simulink model "network_2"  (R2018a)
settings: Solver=VariableStepAuto  StartTime=0.0  StopTime=10.0  RelTol=1e-3
libraries: powerlib x43, fl_lib x2, elec_lib x1
settings Model: Creator=Sadat Zubin Shah  LastModifiedBy=Sadat Zubin Shah

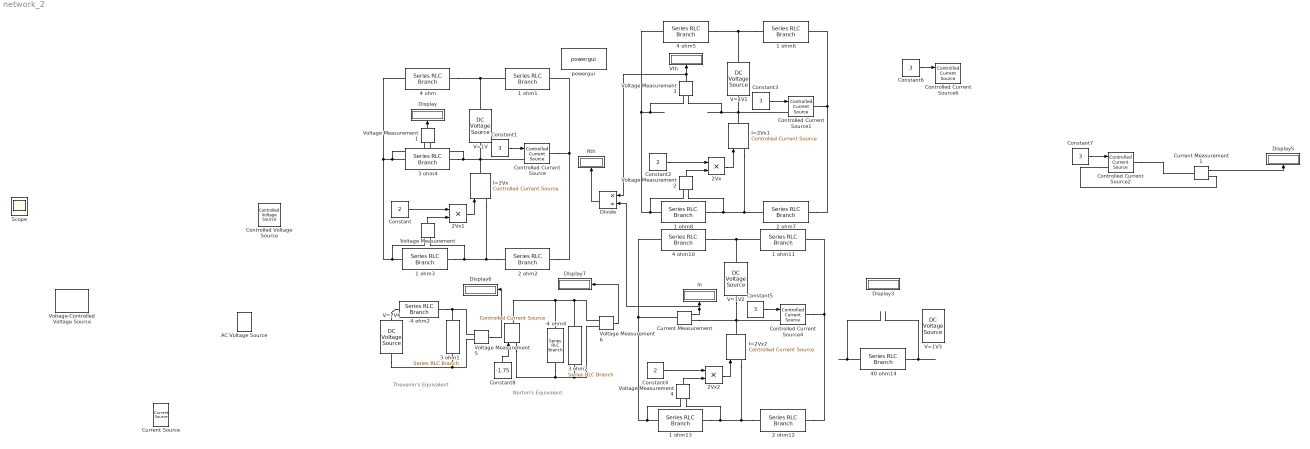
== system network_2 ==
  note: Norton's Equivalent
  note: Thevenin's Equivalent
  " " : powerlib/Electrical Sources/Controlled Current Source  Initialize=off  Source_Type=AC  Amplitude=0  Phase=0  Frequency=0  Measurements=None
  -4 ohm2 : powerlib/Elements/Series RLC Branch  LConnTagsString=__new0  RConnTagsString=__new0  BranchType=R  Resistance=-4  Inductance=1e-3  SetiL0=off  InitialCurrent=0  Capacitance=1e-6  Setx0=off  InitialVoltage=0  Measurements=None
  -4 ohm4 : powerlib/Elements/Series RLC Branch  LConnTagsString=__new0  RConnTagsString=__new0  BranchType=R  Resistance=-4  Inductance=1e-3  SetiL0=off  InitialCurrent=0  Capacitance=1e-6  Setx0=off  InitialVoltage=0  Measurements=None
  1 ohm{1,3,6,8,11,13} (6 alike) : powerlib/Elements/Series RLC Branch  LConnTagsString=__new0  RConnTagsString=__new0  BranchType=R  Resistance=1  Inductance=1e-3  SetiL0=off  InitialCurrent=0  Capacitance=1e-6  Setx0=off  InitialVoltage=0  Measurements=None
  2 ohm12 : powerlib/Elements/Series RLC Branch  LConnTagsString=__new0  RConnTagsString=__new0  BranchType=R  Resistance=2  Inductance=1e-3  SetiL0=off  InitialCurrent=0  Capacitance=1e-6  Setx0=off  InitialVoltage=0  Measurements=None
  2 ohm2 : powerlib/Elements/Series RLC Branch  LConnTagsString=__new0  RConnTagsString=__new0  BranchType=R  Resistance=2  Inductance=1e-3  SetiL0=off  InitialCurrent=0  Capacitance=1e-6  Setx0=off  InitialVoltage=0  Measurements=None
  2 ohm7 : powerlib/Elements/Series RLC Branch  LConnTagsString=__new0  RConnTagsString=__new0  BranchType=R  Resistance=2  Inductance=1e-3  SetiL0=off  InitialCurrent=0  Capacitance=1e-6  Setx0=off  InitialVoltage=0  Measurements=None
  2Vx : Product
  2Vx1 : Product
  2Vx2 : Product
  3 ohm1 : powerlib/Elements/Series RLC Branch  LConnTagsString=__new0  RConnTagsString=__new0  BranchType=R  Resistance=3  Inductance=1e-3  SetiL0=off  InitialCurrent=0  Capacitance=1e-6  Setx0=off  InitialVoltage=0  Measurements=None
  3 ohm2 : powerlib/Elements/Series RLC Branch  LConnTagsString=__new0  RConnTagsString=__new0  BranchType=R  Resistance=3  Inductance=1e-3  SetiL0=off  InitialCurrent=0  Capacitance=1e-6  Setx0=off  InitialVoltage=0  Measurements=None
  3 ohm4 : powerlib/Elements/Series RLC Branch  LConnTagsString=__new0  RConnTagsString=__new0  BranchType=R  Resistance=3  Inductance=1e-3  SetiL0=off  InitialCurrent=0  Capacitance=1e-6  Setx0=off  InitialVoltage=0  Measurements=None
  4 ohm : powerlib/Elements/Series RLC Branch  LConnTagsString=__new0  RConnTagsString=__new0  BranchType=R  Resistance=4  Inductance=1e-3  SetiL0=off  InitialCurrent=0  Capacitance=1e-6  Setx0=off  InitialVoltage=0  Measurements=None
  4 ohm10 : powerlib/Elements/Series RLC Branch  LConnTagsString=__new0  RConnTagsString=__new0  BranchType=R  Resistance=4  Inductance=1e-3  SetiL0=off  InitialCurrent=0  Capacitance=1e-6  Setx0=off  InitialVoltage=0  Measurements=None
  4 ohm5 : powerlib/Elements/Series RLC Branch  LConnTagsString=__new0  RConnTagsString=__new0  BranchType=R  Resistance=4  Inductance=1e-3  SetiL0=off  InitialCurrent=0  Capacitance=1e-6  Setx0=off  InitialVoltage=0  Measurements=None
  40 ohm14 : powerlib/Elements/Series RLC Branch  LConnTagsString=__new0  RConnTagsString=__new0  BranchType=R  Resistance=3  Inductance=1e-3  SetiL0=off  InitialCurrent=0  Capacitance=1e-6  Setx0=off  InitialVoltage=0  Measurements=None
  AC Voltage Source : powerlib/Electrical Sources/AC Voltage Source  Amplitude=100  Phase=0  Frequency=60  SampleTime=0  Measurements=None  BusType=swing  Pref=10e3  Qref=0  Qmin=-inf  Qmax=+inf
  Constant : Constant  Value=2
  Constant{1,3,5..7} (5 alike) : Constant  Value=3
  Constant2 : Constant  Value=2
  Constant4 : Constant  Value=2
  Constant8 : Constant  Value=-1.75
  Controlled Current Source{,1..2,4,6} (5 alike) : powerlib/Electrical Sources/Controlled Current Source  Initialize=off  Source_Type=AC  Amplitude=0  Phase=0  Frequency=0  Measurements=None
  Controlled Voltage Source : fl_lib/Electrical/Electrical Sources/Controlled Voltage Source
  Current Measurement : powerlib/Measurements/Current Measurement  PhasorSimulation=off  OutputType=Complex  PSBequivalent=0
  Current Measurement1 : powerlib/Measurements/Current Measurement  PhasorSimulation=off  OutputType=Complex  PSBequivalent=0
  Current Source : elec_lib/Sources/Current Source  dc_current=0 A  ac_current=0 A  ac_shift=0 rad  ac_frequency=60 Hz  noise_mode=0  PSD=0 A^2/Hz  repeatability=1  auto_seed=3499211588  user_seed=0  sample_time=1e-3 s  i_specify=off  i_priority=None  i=0 A  i_nominal_specify=off  i_nominal_unit=A  i_nominal_value=1  v_specify=off  v_priority=None  v=0 V  v_nominal_specify=off  v_nominal_unit=V  v_nominal_value=1
      settings: SourceProductName=Simscape Electronics  SourceProductBaseCode=SN
  Display{,3,5..7} (5 alike) : Display
  Divide : Product  Inputs=*/
  I=2Vx : powerlib/Electrical Sources/Controlled Current Source  Initialize=off  Source_Type=AC  Amplitude=0  Phase=0  Frequency=0  Measurements=None
  I=2Vx1 : powerlib/Electrical Sources/Controlled Current Source  Initialize=off  Source_Type=AC  Amplitude=0  Phase=0  Frequency=0  Measurements=None
  I=2Vx2 : powerlib/Electrical Sources/Controlled Current Source  Initialize=off  Source_Type=AC  Amplitude=0  Phase=0  Frequency=0  Measurements=None
  In : Display
  Rth : Display
  Scope : Scope
  V=1V : powerlib/Electrical Sources/DC Voltage Source  Amplitude=1  Measurements=None
  V=1V1 : powerlib/Electrical Sources/DC Voltage Source  Amplitude=1  Measurements=None
  V=1V2 : powerlib/Electrical Sources/DC Voltage Source  Amplitude=1  Measurements=None
  V=1V3 : powerlib/Electrical Sources/DC Voltage Source  Amplitude=10  Measurements=None
  V=7V4 : powerlib/Electrical Sources/DC Voltage Source  Amplitude=7  Measurements=None
  Voltage Measurement{,1..6} (7 alike) : powerlib/Measurements/Voltage Measurement  PhasorSimulation=off  OutputType=Complex  PSBequivalent=0
  Voltage-Controlled Voltage Source : fl_lib/Electrical/Electrical Sources/Voltage-Controlled Voltage Source  K=1  v1_specify=off  v1_priority=None  v1=0 V  v1_nominal_specify=off  v1_nominal_unit=V  v1_nominal_value=1  v2_specify=off  v2_priority=None  v2=0 V  v2_nominal_specify=off  v2_nominal_unit=V  v2_nominal_value=1
      settings: SourceProductName=Simscape  SourceProductBaseCode=SS
  Vth : Display
  powergui : powerlib/powergui  Priority=1  SimulationMode=Continuous  SampleTime=50e-6  frequency=60  Iterations=50  frequencyindice=0  Pbase=100e6  ErrMax=1e-4  UnitsV=kV  UnitsW=MW  buscounter=0  FunctionMessages=off  echomessages=off  EnableUseOfTLC=off  CurrentSourceSwitches=off  DisableSnubberDevices=off  DisableRonSwitches=off  DisableVfSwitches=off  DisplayEquations=off  SolverType=Tustin/Backward Euler (TBE)  Interpol=off  ExternalGateDelay=off  methode=off  Ts=100  x0status=blocks  SPID=on  SwTol=0  HookPort=off  RestoreLinks=warning  ResistiveCurrentMeasurement=off  Frange=[0:2:500]  Ylog=off  Xlog=off  ShowGrid=on  save=off  variable=ZData  structure=0  ZoomFFT=off  StartTime=0.0  cycles=1  DisplayStyle=1  fundamental=60  FreqAxis=off  MaxFrequency=1000  frequencyindicesteady=1  RmsSteady=1  display=off
  wires:
  Voltage Measurement/1 -> 2Vx1/2
  Constant/1 -> 2Vx1/1
  2Vx1/1 -> I=2Vx/1
  Constant1/1 -> Controlled Current Source/1
  Voltage Measurement1/1 -> Display/1
  Voltage Measurement3/1 -> Vth/1, Divide/1
  2Vx/1 -> I=2Vx1/1
  Constant2/1 -> 2Vx/1
  Voltage Measurement2/1 -> 2Vx/2
  Voltage Measurement4/1 -> 2Vx2/2
  Constant4/1 -> 2Vx2/1
  2Vx2/1 -> I=2Vx2/1
  Constant5/1 -> Controlled Current Source4/1
  Constant6/1 -> Controlled Current Source6/1
  ? -> Display3/1
  Current Measurement/1 -> Divide/2, In/1
  Divide/1 -> Rth/1
  Constant3/1 -> Controlled Current Source1/1
  Constant7/1 -> Controlled Current Source2/1
  Current Measurement1/1 -> Display5/1
  Voltage Measurement5/1 -> Display6/1
  Constant8/1 -> " "/1
  Voltage Measurement6/1 -> Display7/1
  connections:
  3 ohm4/RConn1 -- Voltage Measurement1/LConn2 -- I=2Vx/RConn1 -- Controlled Current Source/LConn1 -- V=1V/LConn1
  2 ohm2/RConn1 -- Controlled Current Source/RConn1 -- 1 ohm1/RConn1
  2 ohm2/LConn1 -- Voltage Measurement/LConn2 -- 1 ohm3/RConn1 -- I=2Vx/LConn1
  1 ohm3/LConn1 -- Voltage Measurement/LConn1 -- 4 ohm/LConn1 -- Voltage Measurement1/LConn1 -- 3 ohm4/LConn1
  4 ohm/RConn1 -- 1 ohm1/LConn1 -- V=1V/RConn1
  I=2Vx1/RConn1 -- V=1V1/LConn1 -- Controlled Current Source1/LConn1 -- Voltage Measurement3/LConn2
  Voltage Measurement2/LConn2 -- 1 ohm8/RConn1 -- I=2Vx1/LConn1 -- 2 ohm7/LConn1
  Voltage Measurement2/LConn1 -- 1 ohm8/LConn1 -- Voltage Measurement3/LConn1 -- 4 ohm5/LConn1
  1 ohm6/LConn1 -- V=1V1/RConn1 -- 4 ohm5/RConn1
  1 ohm11/RConn1 -- 2 ohm12/RConn1 -- Controlled Current Source4/RConn1
  2 ohm12/LConn1 -- Voltage Measurement4/LConn2 -- 1 ohm13/RConn1 -- I=2Vx2/LConn1
  1 ohm13/LConn1 -- Current Measurement/LConn1 -- 4 ohm10/LConn1 -- Voltage Measurement4/LConn1
  Controlled Current Source4/LConn1 -- Current Measurement/RConn1 -- V=1V2/LConn1 -- I=2Vx2/RConn1
  40 ohm14/RConn1 -- ?
  40 ohm14/LConn1 -- ?
  2 ohm7/RConn1 -- Controlled Current Source1/RConn1 -- 1 ohm6/RConn1
  4 ohm10/RConn1 -- V=1V2/RConn1 -- 1 ohm11/LConn1
  Controlled Current Source2/RConn1 -- Current Measurement1/LConn1
  Current Measurement1/RConn1 -- Controlled Current Source2/LConn1
  V=7V4/RConn1 -- -4 ohm2/LConn1
  -4 ohm2/RConn1 -- Voltage Measurement5/LConn1 -- 3 ohm1/LConn1
  V=7V4/LConn1 -- Voltage Measurement5/LConn2 -- 3 ohm1/RConn1
  Voltage Measurement6/LConn1 -- -4 ohm4/LConn1 -- " "/RConn1 -- 3 ohm2/LConn1
  " "/LConn1 -- -4 ohm4/RConn1 -- Voltage Measurement6/LConn2 -- 3 ohm2/RConn1
